simulink model "cartesian_impedance_control"  (R2025a)
settings: Solver=FixedStepDiscrete  StartTime=0.0  StopTime=inf  FixedStep=0.001  RelTol=1e-3  EnableMultiTasking=on
PreLoadFcn:
  | frs = FrankaRobotSettings;
InitFcn:
  | set_param([gcs,'/End effector y direction translate1'], 'Value', '150');
  | set_param([gcs,'/End effector y direction translate2'], 'Value', '50');
  | set_param([gcs,'/End effector y direction translate'], 'Value', '0');
  | set_param([gcs,'/End effector z direction translate'], 'Value', '0');
undefined symbols (not defined in the file): Effector, End
libraries: franka_toolbox_simulink_library x2, matrix_library x2
settings Model: ExtModeTrigDuration=10000  Creator=vasi_ko  LastModifiedBy=kvasios
settings SolverCC: AlgebraicLoopSolver=TrustRegion
settings DataIOCC: LimitDataPoints=on  SaveFormat=Array  ReturnWorkspaceOutputs=off
settings OptimizationCC: StrengthReduction=on  PassReuseOutputArgsThreshold=0.0  MaxStackSize=64  OptimizeBlockOrder=speed  OptimizationPriority=Speed  OptimizationCustomize=off  MultiThreadedLoops=on  AutoScheduleForLoops=on
settings DebuggingCC: SolverPrmCheckMsg=warning  ParameterTunabilityLossMsg=error  UnconnectedInputMsg=warning  UnconnectedOutputMsg=warning  UnconnectedLineMsg=warning  SFUnexpectedBacktrackingDiag=warning  SFNoUnconditionalDefaultTransitionDiag=warning  SFExecutionAtInitializationDiag=none  ArithmeticOperatorsInVariantConditions=warning
settings HardwareCC: ProdBitPerLong=64.0  ProdHWDeviceType=Intel->x86-64 (Linux 64)
settings ModelReferenceCC: EnableRefExpFcnMdlSchedulingChecks=on  PropagateSignalLabelsOutOfModel=off
settings SFSimCC: SimUseLocalCustomCode=off  MATLABDynamicMemAlloc=off  CustomCodeUndefinedFunction=UseInterfaceOnly  SimTargetLang=C++  SimDLTargetLibrary=mkl-dnn
settings RTWCC: RTWVerbose=off  RTWUseLocalCustomCode=off  BuildConfiguration=Faster Runs  TargetLang=C++  GPUComputeCapability=3.5  DLArmComputeVersion=19.05
settings CodeAppCC: ForceParamTrailComments=on  OperatorAnnotations=on
settings GRTTargetCC: TargetLangStandard=C++11 (ISO)
settings ConfigComp: CovMetricSettings=dw  CovSaveCumulativeToWorkspaceVar=on  CovSaveSingleToWorkspaceVar=on  CovExternalEMLEnable=off  CovSFcnEnable=off

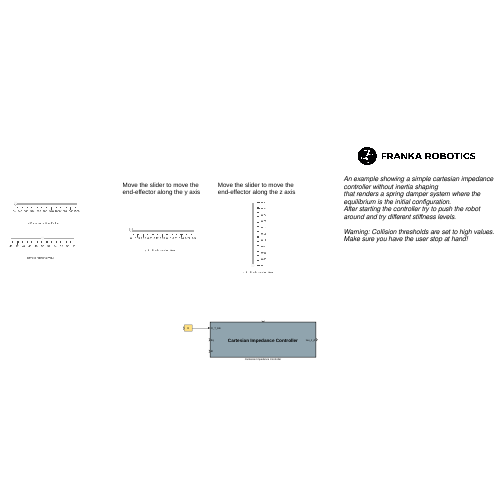
[thumbnail: Simulink's stored preview of the top-level diagram]
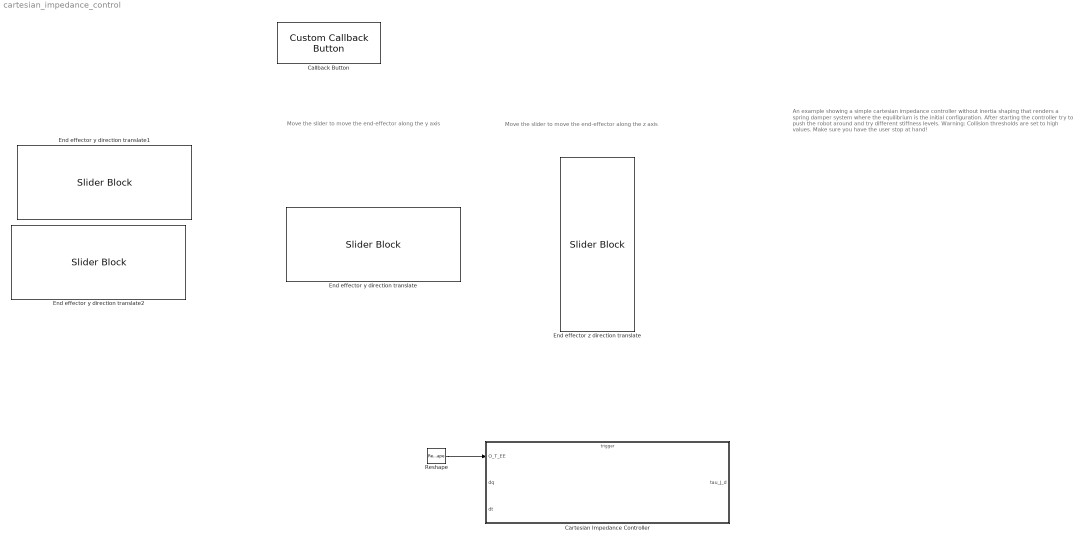
== system cartesian_impedance_control ==
  note: Move the slider to move the end-effector along the y axis
  note: An example showing a simple cartesian impedance controller without inertia shaping
      | that renders a spring damper system where the equilibrium is the initial configuration.
      | After starting the controller try to push the robot around and try different stiffness levels.
      |
      | Warning: Collision thresholds are set to high values. Make sure you have the user stop at hand!
  note: Move the slider to move the end-effector along the z axis
  Callback Button : CustomCallbackButton  Configuration="{\"components\":[{\"name\":\"BackgroundImageComponent\",\"settings\":{\"image\":{\"size\":[0,0],\"src\":\"default\",\"srcOrientation\":\"Right\"},\"position\":[0,0,1,1]}},{\"name\":\"ButtonStateComponent\",\"settings\":{\"buttonType\":\"momentary\",\"clickFcn\":\"set_param([gcs,'\\/End effector y direction translate1'], 'Value', '150');\\nset_param([gcs,'\\/End effector y direction translate2'], 'Value', '50');\\nset_param([gcs,'\\/End effector y direction translate'], 'Value', '0');\\nset_param([gcs,'\\/End effector z direction translate'], 'Value', '0');\",\"onValue\":1,\"position\":[0,0,1,1],\"pressDelay\":\"500\",\"pressFcn\":\"\",\"repeatInterval\":\"0\",\"states\":[{\"horizontalAlignment\":\"center\",\"image\":{\"position\":[0,0,1,1],\"src\":\"default\",\"srcOrientation\":\"Right\"},\"label\":{\"color\":[0.01176470588,0.01176470588,0.01176470588,1],\"icon\":{\"size\":[0,0],\"src\":\"default\",\"srcOrientation\":\"Right\"},\"iconPlacement\":\"left\",\"text\":{\"content\":\"Reset sliders\"}},\"labelOffset\":[0,0],\"verticalAlignment\":\"middle\"},{\"horizontalAlignment\":\"center\",\"image\":{\"position\":[0,0,1,1],\"src\":\"default\",\"srcOrientation\":\"Right\"},\"label\":{\"color\":[0.01176470588,0.01176470588,0.01176470588,1],\"icon\":{\"size\":[0,0],\"src\":\"default\",\"srcOrientation\":\"Right\"},\"iconPlacement\":\"left\",\"text\":{\"content\":\"Reset sliders\"}},\"labelOffset\":[0,0],\"verticalAlignment\":\"middle\"},{\"horizontalAlignment\":\"center\",\"image\":{\"position\":[0,0,1,1],\"src\":\"default\",\"srcOrientation\":\"Right\"},\"label\":{\"color\":[0.01176470588,0.01176470588,0.01176470588,1],\"icon\":{\"size\":[0,0],\"src\":\"default\",\"srcOrientation\":\"Right\"},\"iconPlacement\":\"left\",\"text\":{\"content\":\"Reset sliders\"}},\"labelOffset\":[0,0],\"verticalAlignment\":\"middle\"},{\"horizontalAlignment\":\"center\",\"image\":{\"position\":[0,0,1,1],\"src\":\"default\",\"srcOrientation\":\"Right\"},\"label\":{\"color\":[0.01176470588,0.01176470588,0.01176470588,1],\"icon\":{\"size\":[0,0],\"src\":\"default\",\"srcOrientation\":\"Right\"},\"iconPlacement\":\"left\",\"text\":{\"content\":\"Reset sliders\"}},\"labelOffset\":[0,0],\"verticalAlignment\":\"middle\"}]}},{\"name\":\"ForegroundImageComponent\",\"settings\":{\"image\":{\"size\":[0,0],\"src\":\"default\",\"srcOrientation\":\"Right\"},\"isForeground\":1,\"position\":[0,0,1,1]}}],\"derived\":{\"blockParameters\":{\"AutoActivate\":true,\"ButtonText\":\"Reset sliders\",\"ButtonType\":\"Momentary\",\"ClickFcn\":\"set_param([gcs,'\\/End effector y direction translate1'], 'Value', '150');\\nset_param([gcs,'\\/End effector y direction translate2'], 'Value', '50');\\nset_param([gcs,'\\/End effector y direction translate'], 'Value', '0');\\nset_param([gcs,'\\/End effector z direction translate'], 'Value', '0');\",\"OnValue\":1,\"PressDelay\":\"500\",\"PressFcn\":\"\",\"RepeatInterval\":\"0\",\"fixedAspectRatio\":\"off\"}},\"settings\":{\"BindingType\":\"standalone\",\"autoActivate\":true,\"backgroundColor\":[244,244,244,1],\"backgroundOffset\":0.2,\"backgroundOpacity\":1,\"fixedAspectRatio\":\"off\",\"foregroundColor\":[0.01176470588,0.01176470588,0.01176470588,1],\"migratedFromLegacy\":true,\"useBackgroundColor\":true,\"variant\":\"callback\",\"version\":\"R2025a\"},\"type\":\"Button\"}"  CustomBackgroundColor="{\"color\":[0.9568627451,0.9568627451,0.9568627451],\"show\":true}"
  Cartesian Impedance Controller : Subsystem
      settings: RTWSystemCode=Nonreusable function
      mask Display:
      | disp('{\bf\fontsize{18}Cartesian Impedance Controller}', 'texmode','on');
      | 
      | block_icon('Controller')
      | 
      | port_label('output',1,'tau_J_d');
      | 
      | port_label('input',1,'O_T_EE');
      | port_label('input',2,'dq');
      | port_label('input',3,'dt');
  End effector y direction translate : SliderBlock  LabelPosition=Bottom  ScaleMax=.30
  End effector y direction translate1 : SliderBlock  LabelPosition=Bottom  ScaleMin=100  ScaleMax=1500
  End effector y direction translate2 : SliderBlock  LabelPosition=Bottom  ScaleMin=40  ScaleMax=60
  End effector z direction translate : SliderBlock  LabelPosition=Bottom  ScaleMax=.30
  Reshape : Reshape  OutputDimensionality=Customize  OutputDimensions=[4,4]
  wires:
  Reshape/1 -> Cartesian Impedance Controller/1(O_T_EE)

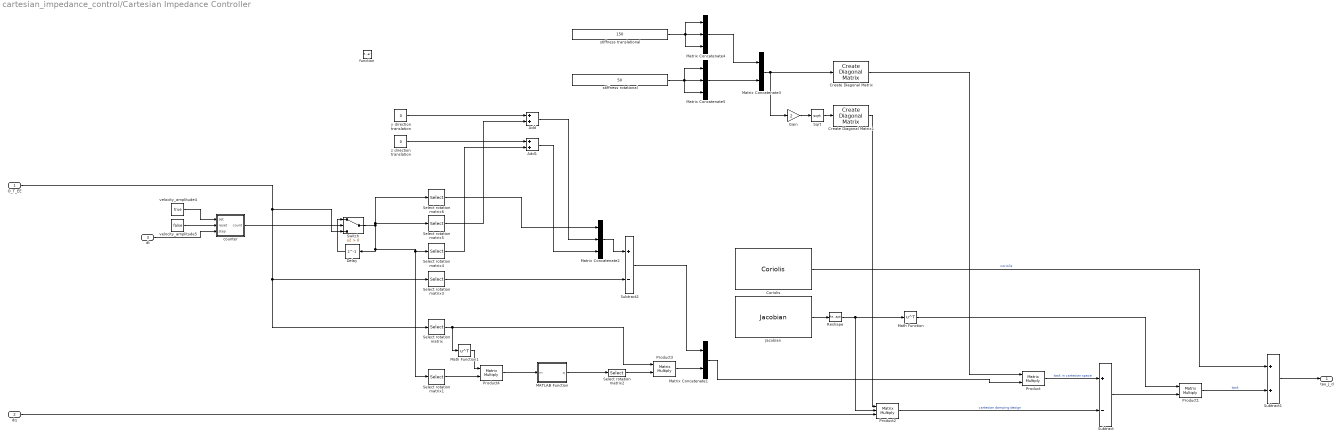
== system cartesian_impedance_control/Cartesian Impedance Controller ==
  O_T_EE : Inport
  dq : Inport  Port=2
  dt : Inport  Port=3
  function : TriggerPort  TriggerType=function-call  VariantControl=(inherit)
  Add : Sum
  Add1 : Sum
  Coriolis : franka_toolbox_simulink_library/Coriolis  robot_ip=frs.robot_ip  robot_state_only=on
      settings: SourceProductName=Franka Robotics Simulink Support Package
  Create Diagonal Matrix : matrix_library/Create Diagonal Matrix
  Create Diagonal Matrix1 : matrix_library/Create Diagonal Matrix
  Delay : Delay  DelayLength=1
  Gain : Gain  Gain=2
  Jacobian : franka_toolbox_simulink_library/Jacobian  robot_ip=frs.robot_ip  jacobian_type=Zero Jabobian  frame=End-Effector  robot_state_only=on
      settings: SourceProductName=Franka Robotics Simulink Support Package
  MATLAB Function : MATLAB Function  TreatAsAtomicUnit=on
  Math Function : Math  Operator=transpose  SignedPower=on
  Math Function1 : Math  Operator=transpose  SignedPower=on
  Matrix Concatenate1 : Concatenate
  Matrix Concatenate2 : Concatenate  NumInputs=3
  Matrix Concatenate3 : Concatenate
  Matrix Concatenate4 : Concatenate  NumInputs=3
  Matrix Concatenate5 : Concatenate  NumInputs=3
  Product{,1,3..4} (4 alike) : Product  Multiplication=Matrix(*)
  Product2 : Product  Inputs=3  Multiplication=Matrix(*)
  Reshape : Reshape  OutputDimensionality=Customize  OutputDimensions=[6,7]
  Select rotation matrix : Selector  NumberOfDimensions=2  InputPortWidth=3  IndexOptions=Index vector (dialog),Index vector (dialog)  Indices=[1,2,3],[1 2 3]  OutputSizes=1
  Select rotation matrix1 : Selector  NumberOfDimensions=2  InputPortWidth=3  IndexOptions=Index vector (dialog),Index vector (dialog)  Indices=[1,2,3],[1 2 3]  OutputSizes=1
  Select rotation matrix2 : Selector  InputPortWidth=4  IndexOptions=Index vector (dialog)  Indices=[2,3,4]  OutputSizes=1
  Select rotation matrix3 : Selector  NumberOfDimensions=2  InputPortWidth=3  IndexOptions=Index vector (dialog),Index vector (dialog)  Indices=[1,2,3],[4]  OutputSizes=1
  Select rotation matrix4 : Selector  NumberOfDimensions=2  InputPortWidth=3  IndexOptions=Index vector (dialog),Index vector (dialog)  Indices=[3],[4]  OutputSizes=1
  Select rotation matrix5 : Selector  NumberOfDimensions=2  InputPortWidth=3  IndexOptions=Index vector (dialog),Index vector (dialog)  Indices=[2],[4]  OutputSizes=1
  Select rotation matrix6 : Selector  NumberOfDimensions=2  InputPortWidth=3  IndexOptions=Index vector (dialog),Index vector (dialog)  Indices=[1],[4]  OutputSizes=1
  Sqrt : Sqrt
  Subtract : Sum  Inputs=+-
  Subtract1 : Sum
  Subtract2 : Sum  Inputs=+-
  Switch : Switch  Criteria=u2 > Threshold  SaturateOnIntegerOverflow=off  InputSameDT=off
  counter : Subsystem
  stiffness rotational : Constant  Value=50  VectorParams1D=off
  stiffness translational : Constant  Value=150  VectorParams1D=off
  velocity_amplitude4 : Constant  Value=true  VectorParams1D=off
  velocity_amplitude5 : Constant  Value=false  VectorParams1D=off
  y direction translation : Constant  Value=0
  z direction translation : Constant  Value=0
  tau_J_d : Outport  VectorParamsAs1DForOutWhenUnconnected=off
  wires:
  Jacobian/1 -> Reshape/1
  Reshape/1 -> Product2/2, Math Function/1
  Math Function/1 -> Product1/1
  Product/1 -> Subtract/1  "task in cartesian space"
  Product2/1 -> Subtract/2  "cartesian damping design"
  Coriolis/1 -> Subtract1/1  "coriolis"
  dq/1 -> Product2/3
  Create Diagonal Matrix1/1 -> Product2/1
  Subtract1/1 -> tau_J_d/1
  Product1/1 -> Subtract1/2  "task"
  O_T_EE/1 -> Select rotation matrix3/1, Select rotation matrix/1, Switch/3
  Switch/1 -> Select rotation matrix6/1, Select rotation matrix5/1, Delay/1, Select rotation matrix4/1, Select rotation matrix1/1
  Select rotation matrix3/1 -> Subtract2/2
  Subtract2/1 -> Matrix Concatenate1/1
  MATLAB Function/1(q) -> Select rotation matrix2/1
  Product4/1 -> MATLAB Function/1(m)
  Subtract/1 -> Product1/2
  Select rotation matrix2/1 -> Product3/2
  Matrix Concatenate1/1 -> Product/2
  Select rotation matrix/1 -> Math Function1/1, Product3/1
  Product3/1 -> Matrix Concatenate1/2
  Select rotation matrix1/1 -> Product4/2
  Math Function1/1 -> Product4/1
  Delay/1 -> Switch/1
  velocity_amplitude4/1 -> counter/1(set)
  counter/1(count) -> Switch/2
  velocity_amplitude5/1 -> counter/2(reset)
  dt/1 -> counter/3(step)
  Matrix Concatenate2/1 -> Subtract2/1
  Select rotation matrix6/1 -> Matrix Concatenate2/1
  y direction translation/1 -> Add/1
  Select rotation matrix5/1 -> Add/2
  Add/1 -> Matrix Concatenate2/2
  z direction translation/1 -> Add1/1
  Select rotation matrix4/1 -> Add1/2
  Add1/1 -> Matrix Concatenate2/3
  Matrix Concatenate3/1 -> Gain/1, Create Diagonal Matrix/1
  Gain/1 -> Sqrt/1
  Sqrt/1 -> Create Diagonal Matrix1/1
  Create Diagonal Matrix/1 -> Product/1
  stiffness translational/1 -> Matrix Concatenate4/1, Matrix Concatenate4/3, Matrix Concatenate4/2
  Matrix Concatenate4/1 -> Matrix Concatenate3/1
  Matrix Concatenate5/1 -> Matrix Concatenate3/2
  stiffness rotational/1 -> Matrix Concatenate5/3, Matrix Concatenate5/1, Matrix Concatenate5/2

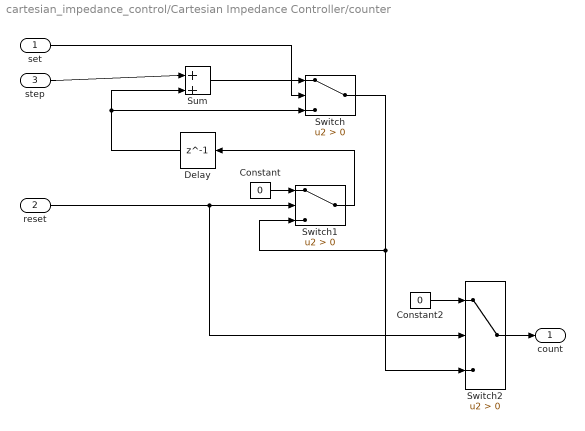
== system cartesian_impedance_control/Cartesian Impedance Controller/counter ==
  set : Inport  OutDataTypeStr=boolean
  reset : Inport  Port=2  OutDataTypeStr=boolean
  step : Inport  Port=3  OutDataTypeStr=double
  Constant : Constant  Value=0  OutDataTypeStr=double
  Constant2 : Constant  Value=0  OutDataTypeStr=double
  Delay : Delay  DelayLength=1  InitialCondition=0
  Sum : Sum  Inputs=|++
  Switch : Switch  Criteria=u2 > Threshold  SaturateOnIntegerOverflow=off  InputSameDT=off
  Switch1 : Switch  Criteria=u2 > Threshold  OutDataTypeStr=double  SaturateOnIntegerOverflow=off  InputSameDT=off
  Switch2 : Switch  Criteria=u2 > Threshold  OutDataTypeStr=double  SaturateOnIntegerOverflow=off  InputSameDT=off
  count : Outport  OutDataTypeStr=double  VectorParamsAs1DForOutWhenUnconnected=off
  wires:
  Switch2/1 -> count/1
  Constant2/1 -> Switch2/1
  Sum/1 -> Switch/1
  set/1 -> Switch/2
  Switch/1 -> Switch1/3, Switch2/3
  step/1 -> Sum/1
  Delay/1 -> Sum/2, Switch/3
  reset/1 -> Switch1/2, Switch2/2
  Constant/1 -> Switch1/1
  Switch1/1 -> Delay/1

== matlab function cartesian_impedance_control/Cartesian Impedance Controller/MATLAB Function ==
  data: m input; q output
function q = rotm2quat(m)

m00 = m(1,1);
m01 = m(1,2);
m02 = m(1,3);

m10 = m(2,1);
m11 = m(2,2);
m12 = m(2,3);

m20 = m(3,1);
m21 = m(3,2);
m22 = m(3,3);

tr = m00 + m11 + m22;

if (tr > 0) 
  S = sqrt(tr+1.0) * 2; % S=4*qw 
  qw = 0.25 * S;
  qx = (m21 - m12) / S;
  qy = (m02 - m20) / S; 
  qz = (m10 - m01) / S; 
elseif ((m00 > m11) && (m00 > m22))
  S = sqrt(1.0 + m00 - m11 - m22) * 2;  %S=4*qx 
  qw = (m21 - m12) / S;
  qx = 0.25 * S;
  qy = (m01 + m10) / S; 
  qz = (m02 + m20) / S; 
elseif (m11 > m22) 
  S = sqrt(1.0 + m11 - m00 - m22) * 2; % S=4*qy
  qw = (m02 - m20) / S;
  qx = (m01 + m10) / S; 
  qy = 0.25 * S;
  qz = (m12 + m21) / S; 
else 
  S = sqrt(1.0 + m22 - m00 - m11) * 2; % S=4*qz
  qw = (m10 - m01) / S;
  qx = (m02 + m20) / S;
  qy = (m12 + m21) / S;
  qz = 0.25 * S;
end

q = [qw,qx,qy,qz]';
